simulink model "Es2home_sim"  (R2018b)
settings: Solver=VariableStepAuto  StartTime=0.0  StopTime=10.0  RelTol=1e-3
libraries: simulink x1
settings Model: Creator=utente  LastModifiedBy=utente

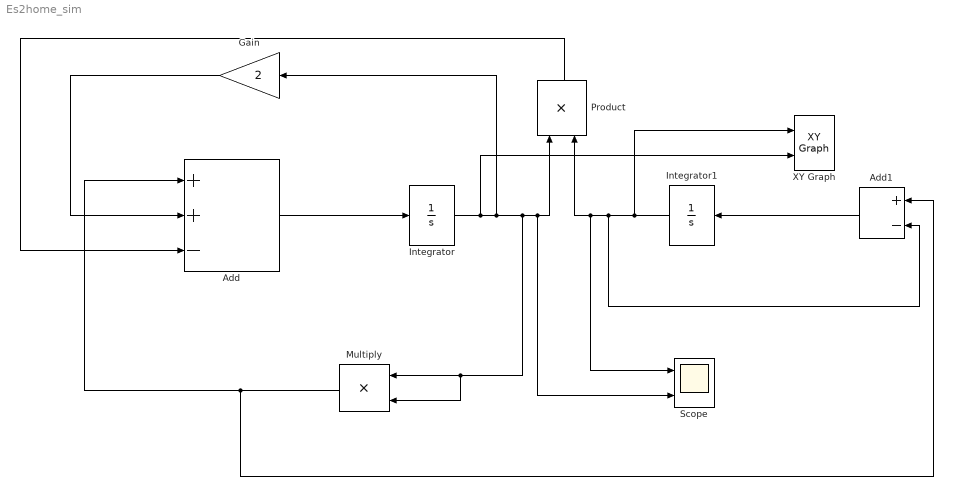
== system Es2home_sim ==
  Add : Sum  Inputs=++-
  Add1 : Sum  Inputs=+-
  Gain : Gain  Gain=2
  Integrator : Integrator  InitialCondition=-1
  Integrator1 : Integrator  InitialCondition=-1
  Multiply : Product
  Product : Product
  Scope : Scope  NumInputPorts=2
  XY Graph : simulink/Sinks/XY Graph  xmin=-5  xmax=5  ymin=-5  ymax=5  st=-1
  wires:
  Add/1 -> Integrator/1
  Integrator/1 -> XY Graph/2, Gain/1, Multiply/2, Multiply/1, Scope/2, Product/1
  Integrator1/1 -> XY Graph/1, Add1/2, Scope/1, Product/2
  Add1/1 -> Integrator1/1
  Multiply/1 -> Add1/1, Add/1
  Gain/1 -> Add/2
  Product/1 -> Add/3
